simulink model "Model_3"  (R2022b)
settings: Solver=ode4  StartTime=0.0  StopTime=10.0  FixedStep=0.01  RelTol=1e-3
settings Model: Creator=student  LastModifiedBy=Jakub
settings DebuggingCC: UnconnectedInputMsg=warning  UnconnectedOutputMsg=warning  UnconnectedLineMsg=warning
settings ModelReferenceCC: EnableRefExpFcnMdlSchedulingChecks=on
settings RTWCC: DLArmComputeVersion=19.05

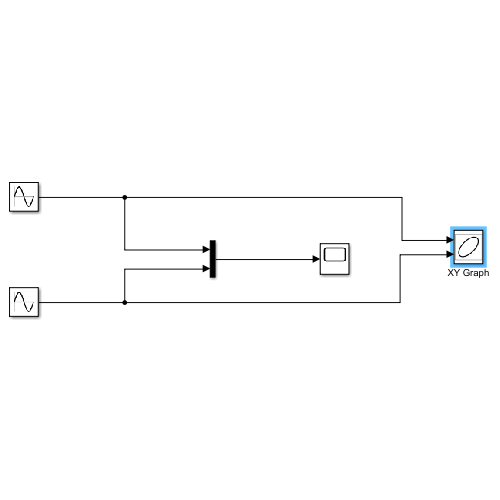
[thumbnail: Simulink's stored preview of the top-level diagram]
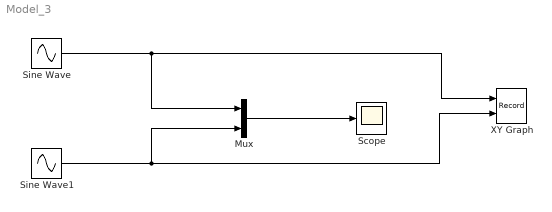
== system Model_3 ==
  Mux : Mux  Inputs=2
  Scope : Scope
  Sine Wave : Sin  Frequency=3  Phase=pi/2  SampleTime=0
  Sine Wave1 : Sin  Frequency=2  SampleTime=0
  XY Graph : Record  FileSettingsInternal="{\"entries\":[{\"content\":{\"excelSettings\":{\"content\":{},\"type\":\"Streamout.ExcelSettings\"}},\"type\":\"Streamout.FileSettingStorage\",\"uuid\":\"87b270df-3282-432e-874c-8ab230b613b2\"}],\"packageUris\":[\"http://schema.mathworks.com/mf0/streamout_blocks/R2020a\"],\"version\":\"1.0\"}"  Layout=[1 1]  SignalsInternal="{\"entries\":[{\"content\":{\"signals\":[{\"content\":{\"blockPath\":[\"Model_3/XY Graph\"],\"channel\":[],\"dimensions\":[1],\"domain\":\"Model_3/XY Graph\",\"lineColor\":\"#a2142f\",\"plots\":[1],\"port\":1,\"sid\":[\"\"],\"signalID\":29,\"signalName\":\"Sine Wave\"},\"type\":\"RecordBlkView.Signal\",\"uuid\":\"4f69513b-7052-433b-a110-ae9b0034d239\"},{\"content\":{\"blockPath\":[\"Model_3/XY Graph\"],\"channel\":[],\"dimensions\":[1],\"domain\":\"Model_3/XY Graph\",\"lineColor\":\"#139fff\",\"plots\":[1],\"port\":2,\"sid\":[\"\"],\"signalID\":33,\"signalName\":\"Sine Wave1\"},\"type\":\"RecordBlkView.Signal\",\"uuid\":\"859754f4-901b-4f1e-a765-dc4d510fdc8d\"}]},\"type\":\"RecordBlkView.InputSignals\",\"uuid\":\"532248e8-4788-4262-8baf-4ab44c8fb37b\"}],\"packageUris\":[\"http://schema.mathworks.com/mf0/streamout_blocks/R2020a\"],\"version\":\"1.0\"}"  VisualizationBindings="{\"xyplotplugin\":{\"info\":[{\"series\":[{\"bindingParametersList\":[{\"parameter\":\"X-Axis\",\"signalID\":29,\"signalName\":\"Sine Wave\"},{\"parameter\":\"Y-Axis\",\"signalID\":33,\"signalName\":\"Sine Wave1\"}],\"seriesID\":16733}],\"subplotID\":1}]}}"  CompatibilityTag=XY  st=-1
  wires:
  Mux/1 -> Scope/1
  Sine Wave1/1 -> XY Graph/2, Mux/2
  Sine Wave/1 -> XY Graph/1, Mux/1
